simulink model "COMM_EXP2_ex"  (Simulink 9.1)
settings: Solver=VariableStepAuto  StartTime=0.0  StopTime=10.0  RelTol=1e-3
undefined symbols (not defined in the file): gcbh, i, rcfiltgaincompat
libraries: dspsrcs4 x4, commsequence2 x2, commfilt2 x2, dspindex x2, commchan3 x1, commrandsrc2 x1, commsink2 x1
settings Model: SuppressorTable=22 serialization::archive 11 0 6 0 0 0 0 0  Creator=zinyy  LastModifiedBy=zinyy
settings DataIOCC: SaveFormat=Dataset
settings OptimizationCC: LifeSpan=auto
settings DebuggingCC: UnderspecifiedInitializationDetection=Simplified  MergeDetectMultiDrivingBlocksExec=error  SFUnexpectedBacktrackingDiag=error  SFNoUnconditionalDefaultTransitionDiag=error  SFExecutionAtInitializationDiag=warning
settings HardwareCC: ProdBitPerPointer=64  ProdBitPerSizeT=64  ProdBitPerPtrDiffT=64  ProdLargestAtomicFloat=Float  ProdIntDivRoundTo=Zero  ProdEndianess=LittleEndian  ProdWordSize=64  ProdHWDeviceType=Intel->x86-64 (Windows64)
settings ModelReferenceCC: PropagateSignalLabelsOutOfModel=on
settings CodeAppCC: StateflowObjectComments=off
settings GRTTargetCC: TargetLangStandard=C99 (ISO)  CombineOutputUpdateFcns=on  GRTInterface=off
settings ConfigComp: CovMetricSettings=dwe  CovHtmlReporting=off  CovSaveCumulativeToWorkspaceVar=off  CovSaveSingleToWorkspaceVar=off  CovExternalEMLEnable=on

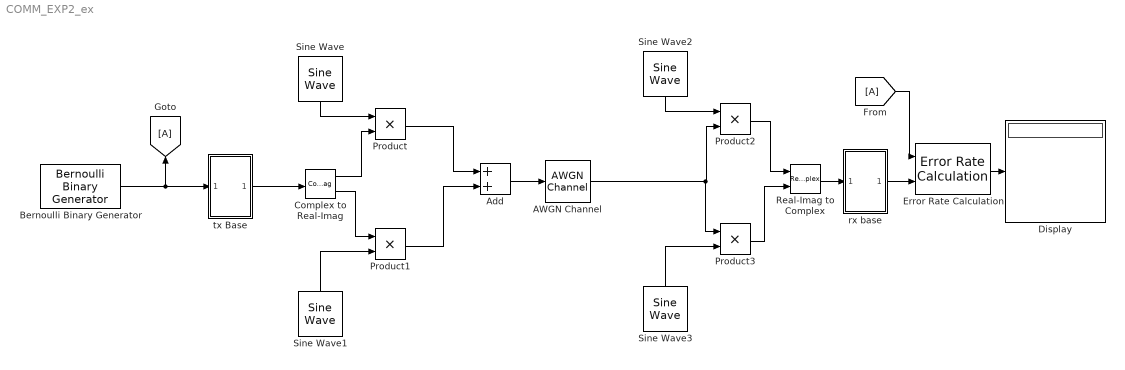
== system COMM_EXP2_ex ==
  AWGN Channel : commchan3/AWGN Channel  InputProcessing=Columns as channels (frame based)  seed=67  noiseMode="Signal to noise ratio  (Eb/No)"  EbNodB=20  EsNodB=10  SNRdB=10  bitsPerSym=2  Ps=1  Tsym=1e-6  variance=1
  Add : Sum
  Bernoulli Binary Generator : commrandsrc2/Bernoulli Binary Generator  P=0.5  seed=61  Ts=5e-7  frameBased=on  sampPerFrame=2000  orient=off  outDataType=double
  Complex to Real-Imag : ComplexToRealImag
  Display : Display
  Error Rate Calculation : commsink2/Error Rate Calculation  N=20  st_delay=0  cp_mode=Entire frame  subframe=[]  PMode=Port  WsName=ErrorVec  RsMode2=off  stop=off  numErr=100  maxBits=1e6
  Product{,1..3} (4 alike) : Product
  Real-Imag to Complex : RealImagToComplex
  Sine Wave : dspsrcs4/Sine Wave  Amplitude=sqrt(2)  Frequency=10e6  Phase=pi/2  SampleMode=Discrete  OutComplex=Real  CompMethod=Trigonometric fcn  TableSize=Speed  SampleTime=1/(40e6)  SamplesPerFrame=4e4  ResetState=Restart at time zero  OutputFrames=off  dataType=double  wordLen=16  udDataType=sfix(16)  fracBitsMode=Best precision  numFracBits=15  OutDataTypeStr=double  LastOutDataTypeStr=double
  Sine Wave1 : dspsrcs4/Sine Wave  Amplitude=-sqrt(2)  Frequency=10e6  Phase=0  SampleMode=Discrete  OutComplex=Real  CompMethod=Trigonometric fcn  TableSize=Speed  SampleTime=1/(40e6)  SamplesPerFrame=4e4  ResetState=Restart at time zero  OutputFrames=off  dataType=double  wordLen=16  udDataType=sfix(16)  fracBitsMode=Best precision  numFracBits=15  OutDataTypeStr=double  LastOutDataTypeStr=double
  Sine Wave2 : dspsrcs4/Sine Wave  Amplitude=sqrt(2)  Frequency=10e6  Phase=pi/2  SampleMode=Discrete  OutComplex=Real  CompMethod=Trigonometric fcn  TableSize=Speed  SampleTime=1/(40e6)  SamplesPerFrame=4e4  ResetState=Restart at time zero  OutputFrames=off  dataType=double  wordLen=16  udDataType=sfix(16)  fracBitsMode=Best precision  numFracBits=15  OutDataTypeStr=double  LastOutDataTypeStr=double
  Sine Wave3 : dspsrcs4/Sine Wave  Amplitude=-sqrt(2)  Frequency=10e6  Phase=0  SampleMode=Discrete  OutComplex=Real  CompMethod=Trigonometric fcn  TableSize=Speed  SampleTime=1/(40e6)  SamplesPerFrame=4e4  ResetState=Restart at time zero  OutputFrames=off  dataType=double  wordLen=16  udDataType=sfix(16)  fracBitsMode=Best precision  numFracBits=15  OutDataTypeStr=double  LastOutDataTypeStr=double
  rx base : Subsystem
  tx Base : Subsystem
  wires:
  Product/1 -> Add/1
  Product3/1 -> Real-Imag to Complex/2
  Sine Wave1/1 -> Product1/2
  Add/1 -> AWGN Channel/1
  Product2/1 -> Real-Imag to Complex/1
  rx base/1(Out1) -> Error Rate Calculation/2
  Complex to Real-Imag/1 -> Product/2
  AWGN Channel/1 -> Product3/1, Product2/2
  [A] -> Error Rate Calculation/1
  Sine Wave2/1 -> Product2/1
  Product1/1 -> Add/2
  Real-Imag to Complex/1 -> rx base/1(In1)
  Sine Wave3/1 -> Product3/2
  Complex to Real-Imag/2 -> Product1/1
  tx Base/1(Out1) -> Complex to Real-Imag/1
  Bernoulli Binary Generator/1 -> tx Base/1(In1), [A]
  Error Rate Calculation/1 -> Display/1
  Sine Wave/1 -> Product/1

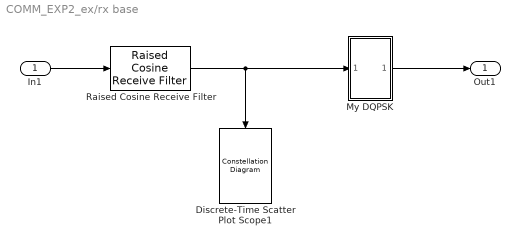
== system COMM_EXP2_ex/rx base ==
  In1 : Inport
  Discrete-Time Scatter Plot Scope1 : ConstellationDiagram  Tag=ScatterPlot
  "My DQPSK " : Subsystem
  Raised Cosine Receive Filter : commfilt2/Raised Cosine Receive Filter  filtType=Square root  R=0.2  filtSpan=2*(5)  N=40  downFactor=40  downOffset=0  filterGain=1/sqrt(40)  InputProcessing=Columns as channels (frame based)  RateOptions=Enforce single-rate processing  framing=Mute  checkCoeff=off  variableName=rcRxFilt  currentFiltSpan=2*(5)  D=5  inputOffset=0  sampMode=Mute  saveAsFlag=0  rateMode=Downsampling  checkGain=Normalized  launchFVT=off  roundingMode=Floor  overflowMode=off  coeffDataTypeStr=Inherit: Same word length as input  coeffMin=[]  coeffMax=[]  coeffLastDataTypeStr=Inherit: Same word length as input  accumDataTypeStr=Inherit: Same as product output  accumLastDataTypeStr=Inherit: Same as product output  outputDataTypeStr=Inherit: Same as accumulator  outputMin=[]  outputMax=[]  outputLastDataTypeStr=Inherit: Same as accumulator
  Out1 : Outport
  wires:
  In1/1 -> Raised Cosine Receive Filter/1
  Raised Cosine Receive Filter/1 -> "My DQPSK "/1(In1), Discrete-Time Scatter Plot Scope1/1
  "My DQPSK "/1(Out1) -> Out1/1

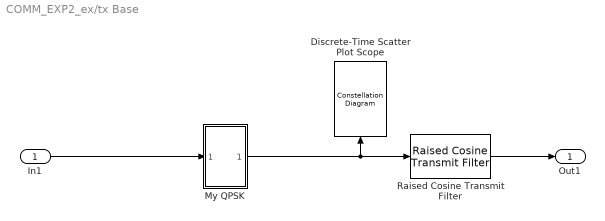
== system COMM_EXP2_ex/tx Base ==
  In1 : Inport
  Discrete-Time Scatter Plot Scope : ConstellationDiagram  Tag=ScatterPlot
  "My QPSK " : Subsystem
  Raised Cosine Transmit Filter : commfilt2/Raised Cosine Transmit Filter  filtType=Square root  R=0.2  filtSpan=2*(5)  N=40  filterGain=(sqrt(40))*rcfiltgaincompat(gcbh)  InputProcessing=Columns as channels (frame based)  RateOptions=Enforce single-rate processing  framing=Mute  checkCoeff=off  variableName=rcTxFilt  checkGain=User-specified  sampMode=Mute  saveAsFlag=0  currentFiltSpan=2*(5)  D=5  launchFVT=off  roundingMode=Floor  overflowMode=off  coeffDataTypeStr=Inherit: Same word length as input  coeffMin=[]  coeffMax=[]  coeffLastDataTypeStr=Inherit: Same word length as input  outputDataTypeStr=Inherit: Same as accumulator  outputMin=[]  outputMax=[]  outputLastDataTypeStr=Inherit: Same as accumulator
  Out1 : Outport
  wires:
  Raised Cosine Transmit Filter/1 -> Out1/1
  "My QPSK "/1(Out1) -> Raised Cosine Transmit Filter/1, Discrete-Time Scatter Plot Scope/1
  In1/1 -> "My QPSK "/1(In1)

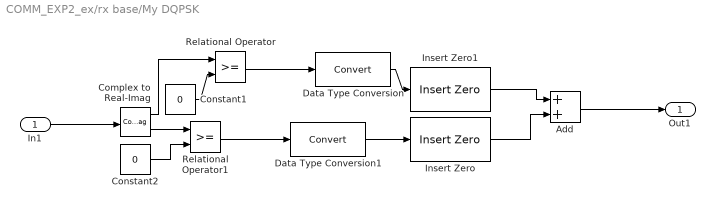
== system COMM_EXP2_ex/rx base/My DQPSK  ==
  In1 : Inport
  Add : Sum
  Complex to Real-Imag : ComplexToRealImag
  Constant1 : Constant  Value=0
  Constant2 : Constant  Value=0
  Data Type Conversion : DataTypeConversion
  Data Type Conversion1 : DataTypeConversion
  Insert Zero : commsequence2/Insert Zero  insertZeroVector=[1 0].'
      settings: SourceProductName=Communications System Toolbox  SourceProductBaseCode=CM
  Insert Zero1 : commsequence2/Insert Zero  insertZeroVector=[0 1].'
      settings: SourceProductName=Communications System Toolbox  SourceProductBaseCode=CM
  Relational Operator : RelationalOperator  OutDataTypeStr=boolean  RndMeth=Simplest
  Relational Operator1 : RelationalOperator  OutDataTypeStr=boolean  RndMeth=Simplest
  Out1 : Outport
  wires:
  Constant2/1 -> Relational Operator1/2
  In1/1 -> Complex to Real-Imag/1
  Add/1 -> Out1/1
  Complex to Real-Imag/2 -> Relational Operator1/1
  Insert Zero1/1 -> Add/1
  Insert Zero/1 -> Add/2
  Relational Operator1/1 -> Data Type Conversion1/1
  Data Type Conversion1/1 -> Insert Zero/1
  Data Type Conversion/1 -> Insert Zero1/1
  Relational Operator/1 -> Data Type Conversion/1
  Constant1/1 -> Relational Operator/2
  Complex to Real-Imag/1 -> Relational Operator/1

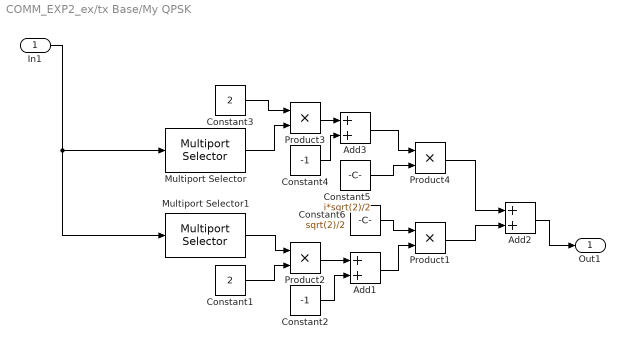
== system COMM_EXP2_ex/tx Base/My QPSK  ==
  In1 : Inport
  Add1 : Sum
  Add2 : Sum
  Add3 : Sum
  Constant1 : Constant  Value=2
  Constant2 : Constant  Value=-1
  Constant3 : Constant  Value=2
  Constant4 : Constant  Value=-1
  Constant5 : Constant  Value=i*sqrt(2)/2
  Constant6 : Constant  Value=sqrt(2)/2
  Multiport Selector : dspindex/Multiport Selector  rowsOrCols=Rows  idxCellArray={1:2:2000}  idxErrMode=Clip Index
  Multiport Selector1 : dspindex/Multiport Selector  rowsOrCols=Rows  idxCellArray={2:2:2000}  idxErrMode=Clip Index
  Product{1..4} (4 alike) : Product
  Out1 : Outport
  wires:
  Constant4/1 -> Add3/2
  Product3/1 -> Add3/1
  Constant1/1 -> Product2/2
  Add3/1 -> Product4/1
  Product4/1 -> Add2/1
  Constant2/1 -> Add1/2
  Multiport Selector1/1 -> Product2/1
  In1/1 -> Multiport Selector1/1, Multiport Selector/1
  Add2/1 -> Out1/1
  Constant3/1 -> Product3/1
  Product2/1 -> Add1/1
  Constant5/1 -> Product4/2
  Multiport Selector/1 -> Product3/2
  Constant6/1 -> Product1/1
  Add1/1 -> Product1/2
  Product1/1 -> Add2/2
